simulink model "sampleModel1590_sub_sub"  (R2023a)
settings: Solver=VariableStepAuto  StartTime=0.0  StopTime=10.0  RelTol=1e-3
libraries: hdlsllib x2, simulink x1
settings Model: Creator=user1  LastModifiedBy=user1
settings OptimizationCC: BlockReduction=off  ConditionallyExecuteInputs=off

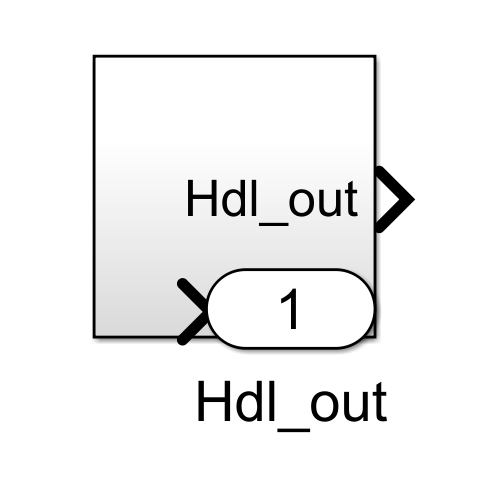
[thumbnail: Simulink's stored preview of the top-level diagram]
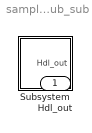
== system sampleModel1590_sub_sub ==
  Subsystem : Subsystem
  Hdl_out : Outport  OutDataTypeStr=uint8

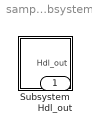
== system sampleModel1590_sub_sub/Subsystem ==
  Subsystem : Subsystem
  Hdl_out : Outport  OutDataTypeStr=uint8

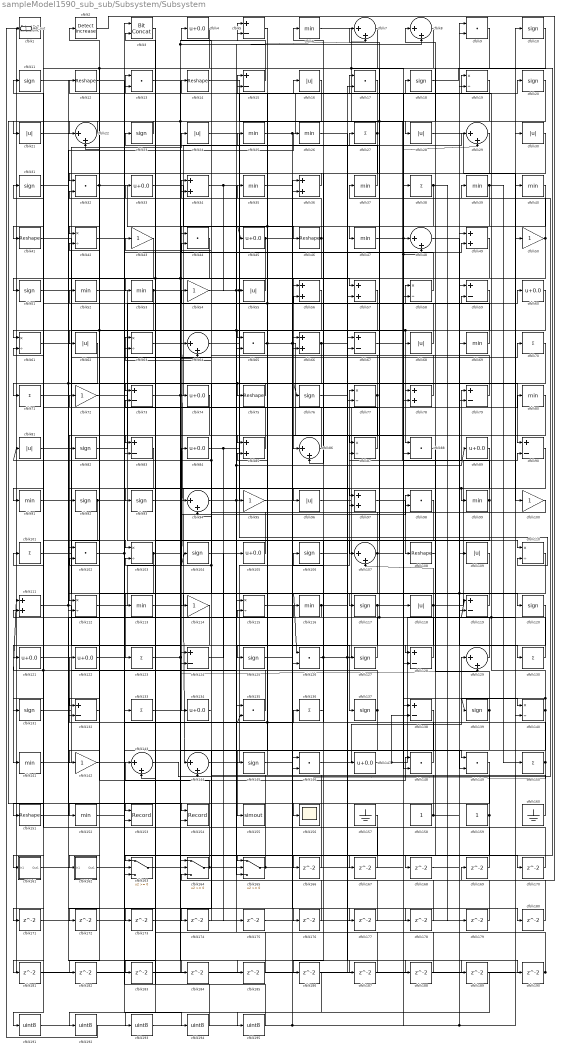
== system sampleModel1590_sub_sub/Subsystem/Subsystem ==
  cfblk1 : hdlsllib/Logic and Bit Operations/Detect Fall Nonpositive  vinit=0  OutDataTypeStr=uint8
  cfblk{10..11,18,20,23,31,51,76,82,92..93,104,106,117,120,125,127,131,137,139,145} (21 alike) : Signum
  cfblk{43,50,54,72,95,100,114,142} (8 alike) : Gain  OutDataTypeStr=uint8
  cfblk{27,38,70..71,101,123,130,133,136,150} (10 alike) : Sum  Inputs=+  OutDataTypeStr=uint8
  cfblk{9,13,17,32,44,65,88,98,102,126,135,146,148..149} (14 alike) : DotProduct  OutDataTypeStr=uint8
  cfblk{19,42,58,61,63,77,87,103,110,112,115,140} (12 alike) : Product  Inputs=*/  OutDataTypeStr=uint8  RndMeth=Zero  SaturateOnIntegerOverflow=on
  cfblk{4,33,45,60,74,84,89,105,121..122,134,147} (12 alike) : Bias  Bias=0.0  SaturateOnIntegerOverflow=off
  cfblk{7..8,22,29,48,64,86,94,107,129,143..144} (12 alike) : Sum  Inputs=|++  OutDataTypeStr=uint8
  cfblk{12,14,41,46,75,108,151} (7 alike) : Reshape
  cfblk{16,21,24,28,30,55,62,68,81,96,109,118} (12 alike) : Abs  OutDataTypeStr=uint8  SaturateOnIntegerOverflow=off
  cfblk{34,36,49,56..57,66,78,85,97,111} (10 alike) : Sum  OutDataTypeStr=uint8
  cfblk{6,25..26,35,37,39..40,47,52..53,69,80,91,99,113,116,141,152} (18 alike) : MinMax  OutDataTypeStr=uint8
  cfblk{5,15,59,67,73,79,83,90,119,124,128,132,138} (13 alike) : Sum  Inputs=+-  OutDataTypeStr=uint8
  cfblk153 : Record  FileSettingsInternal="{\"entries\":[{\"content\":{\"excelSettings\":{\"content\":{},\"type\":\"Streamout.ExcelSettings\"}},\"type\":\"Streamout.FileSettingStorage\",\"uuid\":\"\"}],\"packageUris\":[\"http:\\/\\/schema.mathworks.com\\/mf0\\/streamout_blocks\\/R2020a\"],\"version\":\"1.0\"}"  Layout=[1 1]  SignalsInternal="{\"entries\":[{\"content\":{\"signals\":[{\"content\":{\"blockPath\":[],\"dimensions\":[1],\"domain\":\"\",\"lineColor\":\"#a2142f\",\"plots\":[1],\"port\":1,\"signalID\":28420,\"signalName\":\"cfblk139\"},\"type\":\"RecordBlkView.Signal\",\"uuid\":\"\"},{\"content\":{\"blockPath\":[],\"dimensions\":[1],\"domain\":\"\",\"lineColor\":\"#139fff\",\"plots\":[1],\"port\":2,\"signalID\":28423,\"signalName\":\"cfblk140\"},\"type\":\"RecordBlkView.Signal\",\"uuid\":\"\"}]},\"type\":\"RecordBlkView.InputSignals\",\"uuid\":\"\"}],\"packageUris\":[\"http:\\/\\/schema.mathworks.com\\/mf0\\/streamout_blocks\\/R2020a\"],\"version\":\"1.0\"}"  VisualizationBindings="{\"xyplotplugin\":{\"info\":[{\"series\":[{\"bindingParametersList\":[{\"parameter\":\"X-Axis\",\"signalID\":28420,\"signalName\":\"cfblk139\"},{\"parameter\":\"Y-Axis\",\"signalID\":28423,\"signalName\":\"cfblk140\"}],\"seriesID\":2552}],\"subplotID\":1}]}}"  CompatibilityTag=XY  st=-1
  cfblk154 : Record  FileSettingsInternal="{\"entries\":[{\"content\":{\"excelSettings\":{\"content\":{},\"type\":\"Streamout.ExcelSettings\"}},\"type\":\"Streamout.FileSettingStorage\",\"uuid\":\"\"}],\"packageUris\":[\"http:\\/\\/schema.mathworks.com\\/mf0\\/streamout_blocks\\/R2020a\"],\"version\":\"1.0\"}"  Layout=[1 1]  SignalsInternal="{\"entries\":[{\"content\":{\"signals\":[{\"content\":{\"blockPath\":[],\"dimensions\":[1],\"domain\":\"\",\"lineColor\":\"#a2142f\",\"plots\":[1],\"port\":1,\"signalID\":28412,\"signalName\":\"cfblk22\"},\"type\":\"RecordBlkView.Signal\",\"uuid\":\"\"},{\"content\":{\"blockPath\":[],\"dimensions\":[1],\"domain\":\"\",\"lineColor\":\"#139fff\",\"plots\":[1],\"port\":2,\"signalID\":28415,\"signalName\":\"cfblk50\"},\"type\":\"RecordBlkView.Signal\",\"uuid\":\"\"}]},\"type\":\"RecordBlkView.InputSignals\",\"uuid\":\"\"}],\"packageUris\":[\"http:\\/\\/schema.mathworks.com\\/mf0\\/streamout_blocks\\/R2020a\"],\"version\":\"1.0\"}"  VisualizationBindings="{\"xyplotplugin\":{\"info\":[{\"series\":[{\"bindingParametersList\":[{\"parameter\":\"X-Axis\",\"signalID\":28412,\"signalName\":\"cfblk22\"},{\"parameter\":\"Y-Axis\",\"signalID\":28415,\"signalName\":\"cfblk50\"}],\"seriesID\":8675}],\"subplotID\":1}]}}"  CompatibilityTag=XY  st=-1
  cfblk155 : ToWorkspace  VariableName=simout  SaveFormat=Timeseries  SampleTime=-1
  cfblk156 : Scope
  cfblk157 : Ground
  cfblk158 : Constant  OutDataTypeStr=uint8  SampleTime=-1
  cfblk159 : Constant  OutDataTypeStr=uint8  SampleTime=-1
  cfblk160 : Ground
  cfblk161 : Subsystem
      settings: LibrarySourceBlock=|
      | hdlsllib/Ports &
      | Subsystems/Subsystem
  cfblk162 : Subsystem
      settings: LibrarySourceBlock=|
      | hdlsllib/Ports &
      | Subsystems/Subsystem
  cfblk163 : Switch  OutDataTypeStr=uint8  SaturateOnIntegerOverflow=off  InputSameDT=off
  cfblk164 : Switch  OutDataTypeStr=uint8  SaturateOnIntegerOverflow=off  InputSameDT=off
  cfblk165 : Switch  OutDataTypeStr=uint8  SaturateOnIntegerOverflow=off  InputSameDT=off
  cfblk{166..190} (25 alike) : Delay  SampleTime=1
  cfblk{191..195} (5 alike) : DataTypeConversion  OutDataTypeStr=uint8  SaturateOnIntegerOverflow=off  RndMeth=Floor
  cfblk2 : simulink/Logic and Bit Operations/Detect Increase  vinit=0.0  OutDataTypeStr=uint8
      settings: LibrarySourceBlock=|
      | hdlsllib/Logic and Bit
      | Operations/Detect
      | Increase
  cfblk3 : hdlsllib/Logic and Bit Operations/Bit Concat  numInputs=2
  Hdl_out : Outport  OutDataTypeStr=uint8
  wires:
  cfblk195/1 -> cfblk3/2
  cfblk186/1 -> cfblk195/1
  cfblk194/1 -> cfblk3/1
  cfblk12/1 -> cfblk194/1
  cfblk193/1 -> cfblk88/2, cfblk36/2
  cfblk192/1 -> cfblk1/1
  cfblk189/1 -> cfblk192/1
  cfblk191/1 -> cfblk109/1, cfblk50/1
  cfblk190/1 -> cfblk103/2, Hdl_out/1
  cfblk26/1 -> cfblk190/1
  cfblk163/1 -> cfblk189/1
  cfblk188/1 -> cfblk44/1
  cfblk106/1 -> cfblk188/1
  cfblk187/1 -> cfblk143/1
  cfblk185/1 -> cfblk135/1
  cfblk121/1 -> cfblk185/1
  cfblk184/1 -> cfblk140/2
  cfblk161/1(Out1) -> cfblk184/1
  cfblk183/1 -> cfblk67/1
  cfblk74/1 -> cfblk183/1
  cfblk182/1 -> cfblk128/2
  cfblk181/1 -> cfblk34/2
  cfblk180/1 -> cfblk9/1
  cfblk81/1 -> cfblk180/1
  cfblk179/1 -> cfblk164/3
  cfblk178/1 -> cfblk165/2
  cfblk177/1 -> cfblk115/1
  cfblk125/1 -> cfblk177/1
  cfblk176/1 -> cfblk164/1
  cfblk175/1 -> cfblk17/2
  cfblk174/1 -> cfblk94/2
  cfblk173/1 -> cfblk19/2
  cfblk98/1 -> cfblk173/1
  cfblk172/1 -> cfblk49/1
  cfblk149/1 -> cfblk172/1
  cfblk171/1 -> cfblk58/2
  cfblk57/1 -> cfblk171/1
  cfblk170/1 -> cfblk111/2
  cfblk169/1 -> cfblk36/1
  cfblk2/1 -> cfblk169/1
  cfblk168/1 -> cfblk79/2
  cfblk88/1 -> cfblk168/1
  cfblk167/1 -> cfblk73/2
  cfblk152/1 -> cfblk167/1
  cfblk166/1 -> cfblk32/2
  cfblk35/1 -> cfblk87/1
  cfblk11/1 -> cfblk82/1
  cfblk134/1 -> cfblk54/1, cfblk104/1
  cfblk160/1 -> cfblk63/2
  cfblk165/1 -> cfblk52/1, cfblk81/1, cfblk38/1
  cfblk47/1 -> cfblk148/2, cfblk29/2
  cfblk158/1 -> cfblk59/1, cfblk72/1
  cfblk99/1 -> cfblk156/1, cfblk87/2
  cfblk102/1 -> cfblk80/1, cfblk176/1
  cfblk150/1 -> cfblk144/2, cfblk56/2
  cfblk66/1 -> cfblk132/1, cfblk59/2
  cfblk48/1 -> cfblk130/1
  cfblk86/1 -> cfblk34/1
  cfblk31/1 -> cfblk77/2
  cfblk100/1 -> cfblk97/2
  cfblk58/1 -> cfblk44/2
  cfblk136/1 -> cfblk106/1
  cfblk45/1 -> cfblk102/1, cfblk178/1
  cfblk95/1 -> cfblk127/1
  cfblk39/1 -> cfblk67/2, cfblk150/1
  cfblk151/1 -> cfblk116/1
  cfblk123/1 -> cfblk149/1, cfblk98/2
  cfblk90/1 -> cfblk112/2
  cfblk80/1 -> cfblk125/1
  cfblk3/1 -> cfblk193/1
  cfblk10/1 -> cfblk151/1
  cfblk162/1(Out1) -> cfblk148/1
  cfblk133/1 -> cfblk5/2, cfblk8/2
  cfblk29/1 -> cfblk86/2
  cfblk145/1 -> cfblk66/1
  cfblk15/1 -> cfblk5/1
  cfblk107/1 -> cfblk20/1, cfblk48/2, cfblk13/1, cfblk145/1
  cfblk157/1 -> cfblk163/2
  cfblk53/1 -> cfblk181/1, cfblk182/1, cfblk64/2
  cfblk56/1 -> cfblk83/1
  cfblk7/1 -> cfblk22/2
  cfblk79/1 -> cfblk25/1
  cfblk16/1 -> cfblk93/1
  cfblk9/1 -> cfblk28/1
  cfblk13/1 -> cfblk65/2
  cfblk85/1 -> cfblk42/2
  cfblk139/1 -> cfblk153/1, cfblk8/1
  cfblk69/1 -> cfblk15/2, cfblk33/1
  cfblk43/1 -> cfblk61/1
  cfblk97/1 -> cfblk108/1
  cfblk140/1 -> cfblk12/1, cfblk119/1, cfblk139/1, cfblk153/2
  cfblk131/1 -> cfblk94/1
  cfblk76/1 -> cfblk147/1
  cfblk164/1 -> cfblk18/1, cfblk102/2
  cfblk119/1 -> cfblk113/1
  cfblk28/1 -> cfblk100/1
  cfblk1/1 -> cfblk191/1
  cfblk72/1 -> cfblk97/1
  cfblk128/1 -> cfblk16/1, cfblk7/1
  cfblk8/1 -> cfblk107/1
  cfblk112/1 -> cfblk84/1
  cfblk30/1 -> cfblk56/1
  cfblk91/1 -> cfblk117/1
  cfblk138/1 -> cfblk155/1
  cfblk5/1 -> cfblk65/1
  cfblk130/1 -> cfblk101/1
  cfblk17/1 -> cfblk92/1
  cfblk87/1 -> cfblk11/1
  cfblk141/1 -> cfblk95/1
  cfblk104/1 -> cfblk146/2
  cfblk89/1 -> cfblk128/1, cfblk99/1
  cfblk50/1 -> cfblk154/2, cfblk71/1, cfblk37/1
  cfblk49/1 -> cfblk143/2
  cfblk37/1 -> cfblk14/1
  cfblk34/1 -> cfblk126/2, cfblk55/1
  cfblk126/1 -> cfblk10/1, cfblk149/2, cfblk186/1
  cfblk4/1 -> cfblk62/1, cfblk121/1
  cfblk148/1 -> cfblk135/2, cfblk85/2
  cfblk44/1 -> cfblk73/1, cfblk91/1
  cfblk129/1 -> cfblk6/1
  cfblk40/1 -> cfblk64/1
  cfblk62/1 -> cfblk161/1(In1)
  cfblk75/1 -> cfblk74/1
  cfblk116/1 -> cfblk57/2, cfblk115/2
  cfblk68/1 -> cfblk31/1
  cfblk115/1 -> cfblk146/1
  cfblk84/1 -> cfblk30/1, cfblk175/1
  cfblk117/1 -> cfblk163/1, cfblk29/1
  cfblk73/1 -> cfblk9/2, cfblk129/2
  cfblk101/1 -> cfblk70/1
  cfblk71/1 -> cfblk133/1
  cfblk83/1 -> cfblk152/1
  cfblk105/1 -> cfblk63/1
  cfblk111/1 -> cfblk124/2, cfblk26/1
  cfblk120/1 -> cfblk124/1
  cfblk55/1 -> cfblk51/1
  cfblk65/1 -> cfblk138/1, cfblk170/1, cfblk35/1
  cfblk159/1 -> cfblk15/1, cfblk163/3
  cfblk96/1 -> cfblk69/1
  cfblk77/1 -> cfblk112/1, cfblk23/1
  cfblk142/1 -> cfblk136/1
  cfblk127/1 -> cfblk4/1
  cfblk82/1 -> cfblk60/1
  cfblk63/1 -> cfblk58/1
  cfblk64/1 -> cfblk90/1
  cfblk18/1 -> cfblk165/1
  cfblk67/1 -> cfblk140/1
  cfblk109/1 -> cfblk126/1, cfblk119/2
  cfblk38/1 -> cfblk45/1, cfblk85/1, cfblk179/1
  cfblk19/1 -> cfblk41/1, cfblk47/1
  cfblk70/1 -> cfblk75/1, cfblk114/1
  cfblk122/1 -> cfblk49/2
  cfblk135/1 -> cfblk111/1, cfblk61/2
  cfblk21/1 -> cfblk53/1
  cfblk61/1 -> cfblk68/1
  cfblk27/1 -> cfblk22/1, cfblk83/2
  cfblk118/1 -> cfblk137/1, cfblk90/2, cfblk107/2
  cfblk42/1 -> cfblk57/1
  cfblk46/1 -> cfblk86/1, cfblk13/2
  cfblk147/1 -> cfblk40/1, cfblk138/2
  cfblk132/1 -> cfblk2/1
  cfblk32/1 -> cfblk134/1, cfblk142/1
  cfblk143/1 -> cfblk39/1
  cfblk92/1 -> cfblk131/1, cfblk166/1
  cfblk23/1 -> cfblk21/1
  cfblk78/1 -> cfblk43/1
  cfblk20/1 -> cfblk42/1, cfblk164/2
  cfblk103/1 -> cfblk162/1(In1), cfblk120/1
  cfblk144/1 -> cfblk77/1
  cfblk36/1 -> cfblk32/1
  cfblk113/1 -> cfblk98/1
  cfblk110/1 -> cfblk123/1
  cfblk146/1 -> cfblk129/1
  cfblk93/1 -> cfblk96/1
  cfblk22/1 -> cfblk154/1
  cfblk54/1 -> cfblk17/1, cfblk66/2, cfblk78/2
  cfblk59/1 -> cfblk144/1, cfblk165/3
  cfblk108/1 -> cfblk122/1
  cfblk51/1 -> cfblk76/1, cfblk187/1
  cfblk6/1 -> cfblk118/1, cfblk48/1
  cfblk41/1 -> cfblk103/1
  cfblk114/1 -> cfblk141/1
  cfblk124/1 -> cfblk105/1
  cfblk33/1 -> cfblk46/1
  cfblk25/1 -> cfblk19/1, cfblk78/1
  cfblk14/1 -> cfblk79/1
  cfblk94/1 -> cfblk89/1, cfblk7/2, cfblk27/1
  cfblk137/1 -> cfblk24/1, cfblk174/1
  cfblk24/1 -> cfblk110/2
  cfblk52/1 -> cfblk110/1
  cfblk60/1 -> cfblk88/1, cfblk132/2

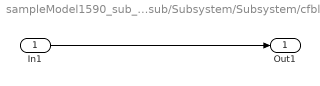
== system sampleModel1590_sub_sub/Subsystem/Subsystem/cfblk161 ==
  In1 : Inport
  Out1 : Outport
  wires:
  In1/1 -> Out1/1

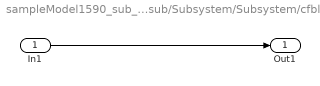
== system sampleModel1590_sub_sub/Subsystem/Subsystem/cfblk162 ==
  In1 : Inport
  Out1 : Outport
  wires:
  In1/1 -> Out1/1
